simulink model "omnibundle_centr_joint"  (R2018b)
settings: Solver=ode23t  StartTime=0.0  StopTime=9  RelTol=1e-3
values from neighbouring files (symbols this model uses):
  ddqv = ddt(ddt(qv,dts),dts)    [main.m]    (also in traj_planning.m)
  dq0 = [0 0 0]'    [main.m]
  dqv = ddt(qv,dts)    [main.m]    (also in traj_planning.m)
  K_D = diag(repmat(2*zeta*wn,3,1))    [main.m]
  K_P = diag(repmat(wn^2,3,1))    [main.m]
  q0 = qs(1,2:4)'    [main.m]
  qv = []    [main.m]    (also in traj_planning.m)
  tau_d = [0;0.1;0]    [main.m]
  tv = 0:dts:qs(end,1)    [main.m]    (also in traj_planning.m)
settings Model: Creator=lucas  LastModifiedBy=lucas
settings SolverCC: ZeroCrossAlgorithm=Adaptive
settings DebuggingCC: IgnoredZcDiagnostic=none

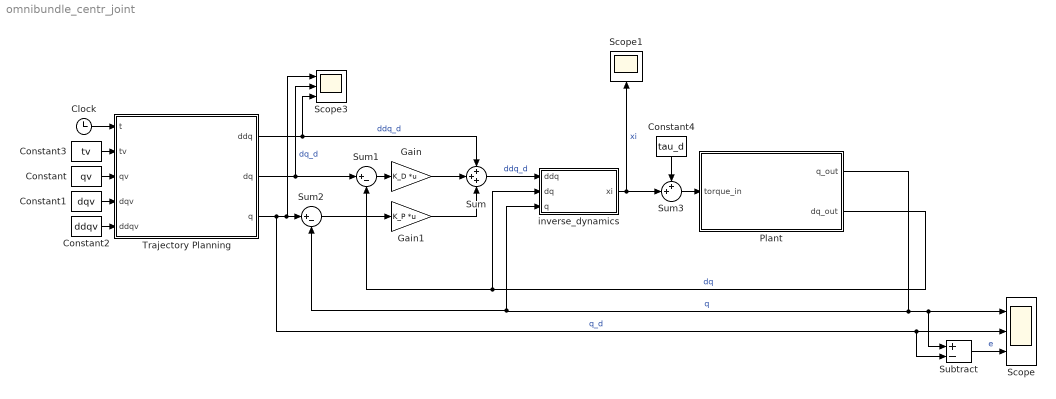
== system omnibundle_centr_joint ==
  Clock : Clock
  Constant : Constant  Value=qv
  Constant1 : Constant  Value=dqv
  Constant2 : Constant  Value=ddqv
  Constant3 : Constant  Value=tv
  Constant4 : Constant  Value=tau_d
  Gain : Gain  Gain=K_D  Multiplication=Matrix(K*u)
  Gain1 : Gain  Gain=K_P  Multiplication=Matrix(K*u)
  Plant : Subsystem
  Scope : Scope  NumInputPorts=3
  Scope1 : Scope
  Scope3 : Scope  NumInputPorts=3
  Subtract : Sum  Inputs=+-
  Sum : Sum  Inputs=+++
  Sum1 : Sum  Inputs=|+-
  Sum2 : Sum  Inputs=|+-
  Sum3 : Sum  Inputs=++|
  Trajectory Planning : MATLAB Function  TreatAsAtomicUnit=on
  inverse_dynamics : MATLAB Function  TreatAsAtomicUnit=on
  wires:
  Subtract/1 -> Scope/3  "e"
  Trajectory Planning/3(q) -> Scope3/1, Sum2/1, Subtract/2, Scope/2  "q_d"
  Clock/1 -> Trajectory Planning/1(t)
  Plant/1(q_out) -> Subtract/1, Scope/1, inverse_dynamics/3(q), Sum2/2  "q"
  Sum/1 -> inverse_dynamics/1(ddq)  "ddq_d"
  Trajectory Planning/1(ddq) -> Sum/1, Scope3/3  "ddq_d"
  Trajectory Planning/2(dq) -> Sum1/1, Scope3/2  "dq_d"
  Sum1/1 -> Gain/1
  Gain/1 -> Sum/2
  Sum2/1 -> Gain1/1
  Gain1/1 -> Sum/3
  inverse_dynamics/1(xi) -> Sum3/2, Scope1/1  "xi"
  Plant/2(dq_out) -> Sum1/2, inverse_dynamics/2(dq)  "dq"
  Constant1/1 -> Trajectory Planning/4(dqv)
  Constant2/1 -> Trajectory Planning/5(ddqv)
  Constant/1 -> Trajectory Planning/3(qv)
  Constant3/1 -> Trajectory Planning/2(tv)
  Sum3/1 -> Plant/1(torque_in)
  Constant4/1 -> Sum3/1

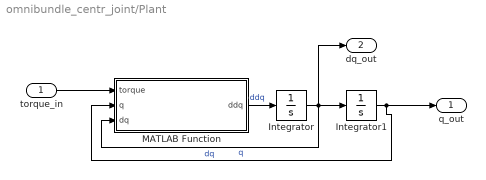
== system omnibundle_centr_joint/Plant ==
  torque_in : Inport
  Integrator : Integrator  InitialCondition=dq0
  Integrator1 : Integrator  InitialCondition=q0
  MATLAB Function : MATLAB Function  TreatAsAtomicUnit=on
  q_out : Outport
  dq_out : Outport  Port=2
  wires:
  MATLAB Function/1(ddq) -> Integrator/1  "ddq"
  Integrator/1 -> dq_out/1, MATLAB Function/3(dq), Integrator1/1  "dq"
  Integrator1/1 -> q_out/1, MATLAB Function/2(q)  "q"
  torque_in/1 -> MATLAB Function/1(torque)

== matlab function omnibundle_centr_joint/inverse_dynamics ==
  data: ddq input; dq input; q input; xi output
function xi = inv_dyn(ddq,dq,q)

xi = inv_dyn_omni_bundle_fun(9.8, q, dq, ddq);

== matlab function omnibundle_centr_joint/Plant/MATLAB Function ==
  data: torque input; q input; dq input; ddq output
function ddq = omnibundle_dyn(torque,q,dq)
    
    ddq = dyn_omni_bundle_fun(9.8, q, dq, torque);

== matlab function omnibundle_centr_joint/Trajectory Planning ==
  data: t input; tv input; ddq output; dq output; q output; qv input; dqv input; ddqv input
function [ddq,dq,q] = trajectory_planning(t, tv, qv, dqv, ddqv)

    if t > tv(end-2)
        t = tv(end-2);
    end

    q = interp1(tv',qv',t)';
    dq = interp1(tv(1:end-1)',dqv',t)';
    ddq = interp1(tv(1:end-2)',ddqv',t)';
